simulink model "M1_P3_A_1"  (R2023a)
settings: Solver=VariableStepAuto  StartTime=0.0  StopTime=1.5  RelTol=1e-3
undefined symbols (not defined in the file): f_eff, J_eff, Kb, Ktn, L, R
settings Model: Creator=azzam  LastModifiedBy=azzam

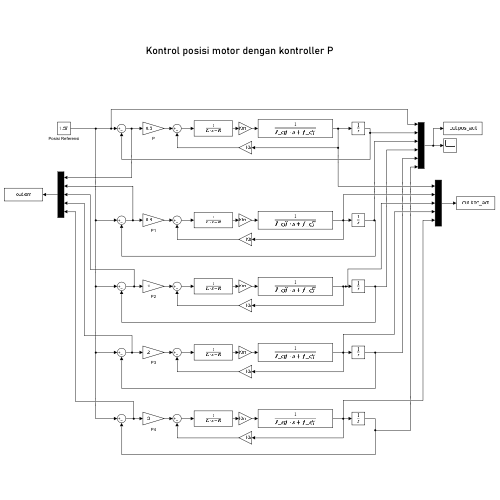
[thumbnail: Simulink's stored preview of the top-level diagram]
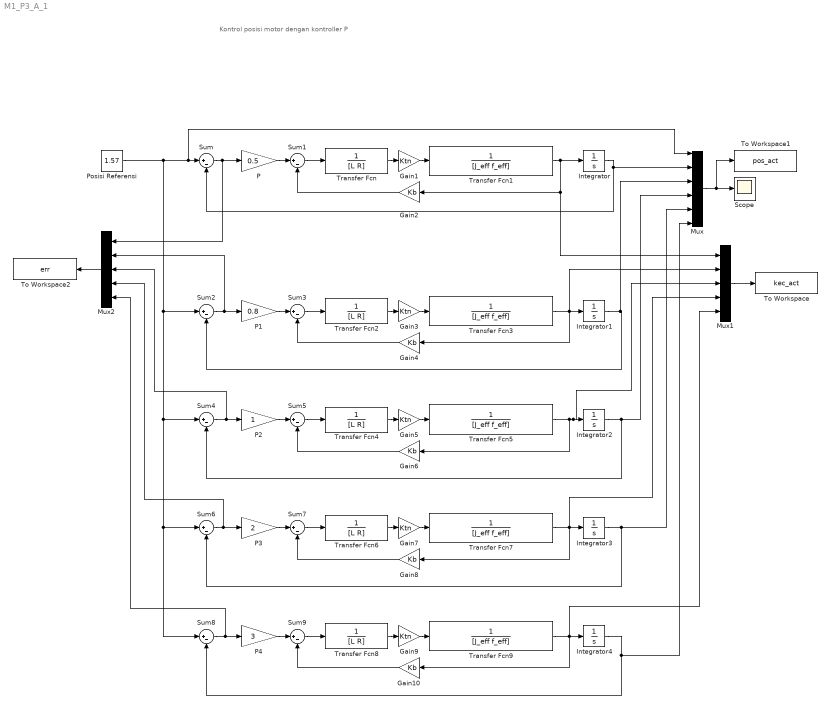
== system M1_P3_A_1 ==
  note: Kontrol posisi motor dengan kontroller P
  Gain{1,3,5,7,9} (5 alike) : Gain  Gain=Ktn
  Gain{2,4,6,8,10} (5 alike) : Gain  Gain=Kb
  Integrator{,1..4} (5 alike) : Integrator
  Mux : Mux  Inputs=6
  Mux1 : Mux  Inputs=5
  Mux2 : Mux  Inputs=5
  P : Gain  Gain=0.5
  P1 : Gain  Gain=0.8
  P2 : Gain
  P3 : Gain  Gain=2
  P4 : Gain  Gain=3
  Posisi Referensi : Constant  Value=1.57
  Scope : Scope
  Sum{,1..9} (10 alike) : Sum  Inputs=|+-
  To Workspace : ToWorkspace  VariableName=kec_act  SaveFormat=Timeseries  SampleTime=-1
  To Workspace1 : ToWorkspace  VariableName=pos_act  SaveFormat=Timeseries  SampleTime=-1
  To Workspace2 : ToWorkspace  VariableName=err  SaveFormat=Timeseries  SampleTime=-1
  Transfer Fcn{,2,4,6,8} (5 alike) : TransferFcn  Denominator=[L R]
  Transfer Fcn{1,3,5,7,9} (5 alike) : TransferFcn  Denominator=[J_eff f_eff]
  wires:
  Posisi Referensi/1 -> Sum8/1, Sum6/1, Sum4/1, Sum2/1, Mux/1, Sum/1
  Sum/1 -> Mux2/1, P/1
  P/1 -> Sum1/1
  Sum1/1 -> Transfer Fcn/1
  Transfer Fcn/1 -> Gain1/1
  Gain1/1 -> Transfer Fcn1/1
  Transfer Fcn1/1 -> Mux1/1, Gain2/1, Integrator/1
  Gain2/1 -> Sum1/2
  Integrator/1 -> Sum/2, Mux/2
  Mux/1 -> To Workspace1/1, Scope/1
  Mux1/1 -> To Workspace/1
  Mux2/1 -> To Workspace2/1
  Integrator1/1 -> Mux/3, Sum2/2
  Transfer Fcn2/1 -> Gain3/1
  Transfer Fcn3/1 -> Gain4/1, Mux1/2, Integrator1/1
  Gain3/1 -> Transfer Fcn3/1
  Sum2/1 -> Mux2/2, P1/1
  P1/1 -> Sum3/1
  Gain4/1 -> Sum3/2
  Sum3/1 -> Transfer Fcn2/1
  Sum5/1 -> Transfer Fcn4/1
  Transfer Fcn4/1 -> Gain5/1
  Transfer Fcn5/1 -> Mux1/3, Integrator2/1, Gain6/1
  P2/1 -> Sum5/1
  Gain5/1 -> Transfer Fcn5/1
  Sum4/1 -> Mux2/3, P2/1
  Integrator2/1 -> Mux/4, Sum4/2
  Gain6/1 -> Sum5/2
  Sum7/1 -> Transfer Fcn6/1
  Transfer Fcn6/1 -> Gain7/1
  Transfer Fcn7/1 -> Mux1/4, Gain8/1, Integrator3/1
  P3/1 -> Sum7/1
  Gain7/1 -> Transfer Fcn7/1
  Sum6/1 -> Mux2/4, P3/1
  Integrator3/1 -> Mux/5, Sum6/2
  Gain8/1 -> Sum7/2
  Sum9/1 -> Transfer Fcn8/1
  Transfer Fcn8/1 -> Gain9/1
  Transfer Fcn9/1 -> Mux1/5, Gain10/1, Integrator4/1
  P4/1 -> Sum9/1
  Gain9/1 -> Transfer Fcn9/1
  Sum8/1 -> Mux2/5, P4/1
  Integrator4/1 -> Mux/6, Sum8/2
  Gain10/1 -> Sum9/2
